simulink model "scratch_luenberger"  (R2020b)
settings: Solver=VariableStepAuto  StartTime=0.0  StopTime=36000  RelTol=1e-3
values from neighbouring files (symbols this model uses):
  F_k = k*[1/theta2 -theta3 -theta3]    [script1.m]
  theta1 = 0.21    [script1.m]
  theta2 = 17.5    [script1.m]
undefined symbols (not defined in the file or in its folder): A_zoh, B_zoh, C_zoh, L
settings Model: Creator=Francesco  LastModifiedBy=Francesco

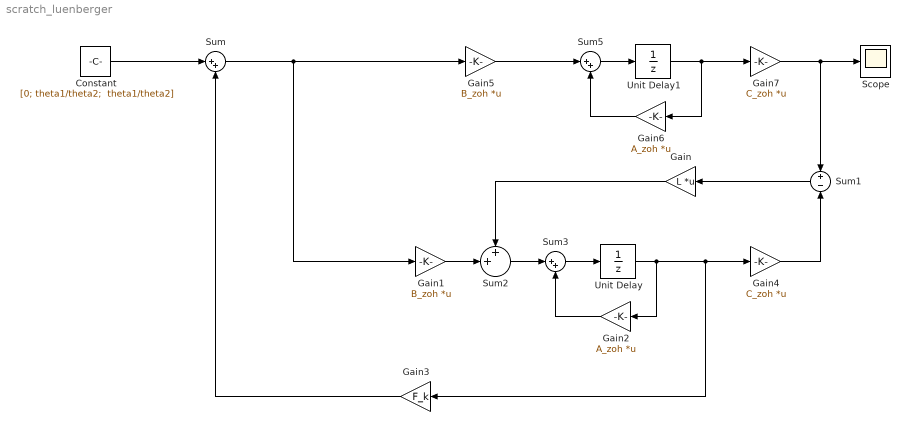
== system scratch_luenberger ==
  Constant : Constant  Value="[0; theta1/theta2;  theta1/theta2]"
  Gain : Gain  Gain=L  Multiplication=Matrix(K*u)
  Gain1 : Gain  Gain=B_zoh  Multiplication=Matrix(K*u)
  Gain2 : Gain  Gain=A_zoh  Multiplication=Matrix(K*u)
  Gain3 : Gain  Gain=F_k
  Gain4 : Gain  Gain=C_zoh  Multiplication=Matrix(K*u)
  Gain5 : Gain  Gain=B_zoh  Multiplication=Matrix(K*u)
  Gain6 : Gain  Gain=A_zoh  Multiplication=Matrix(K*u)
  Gain7 : Gain  Gain=C_zoh  Multiplication=Matrix(K*u)
  Scope : Scope
  Sum : Sum  Inputs=|++
  Sum1 : Sum  Inputs=+|-
  Sum2 : Sum  Inputs=++|
  Sum3 : Sum  Inputs=|++
  Sum5 : Sum  Inputs=|++
  Unit Delay : UnitDelay  SampleTime=-1  HasFrameUpgradeWarning=on
  Unit Delay1 : UnitDelay  SampleTime=-1  HasFrameUpgradeWarning=on
  wires:
  Sum1/1 -> Gain/1
  Gain3/1 -> Sum/2
  Gain4/1 -> Sum1/2
  Sum/1 -> Gain5/1, Gain1/1
  Sum3/1 -> Unit Delay/1
  Gain2/1 -> Sum3/2
  Sum2/1 -> Sum3/1
  Gain1/1 -> Sum2/2
  Gain/1 -> Sum2/1
  Constant/1 -> Sum/1
  Sum5/1 -> Unit Delay1/1
  Gain6/1 -> Sum5/2
  Gain5/1 -> Sum5/1
  Unit Delay1/1 -> Gain7/1, Gain6/1
  Gain7/1 -> Sum1/1, Scope/1
  Unit Delay/1 -> Gain2/1, Gain3/1, Gain4/1
